simulink model "rsim_param_tuning"  (Simulink 5.0)
settings: Solver=VariableStepDiscrete  StartTime=0.0  StopTime=48  FixedStep=1  RelTol=1e-3
PreLoadFcn:
  | clear;INC=uint8(1);LIMIT=uint8(16);K=int32(2);RESET=uint8(0);
StartFcn:
  | platform_finder('')
settings Model: CovMetricSettings=d  Creator=pszpak  LastModifiedBy=dcabral  ExtModeTrigMode=oneshot  ExtModeArmWhenConnect=off  ExtModeAutoUpdateStatusClock=off  TunableVars=INC,LIMIT,RESET,K  TunableVarsStorageClass=ExportedGlobal,ExportedGlobal,ExportedGlobal,ExportedGlobal  TunableVarsTypeQualifier=,,,  BufferReuse=off  SaveFormat=StructureWithTime  LimitDataPoints=off  IntegerOverflowMsg=none  RTWInlineParameters=on  ProdHWWordLengths=8,32,16,32  RTWSystemTargetFile=rsim.tlc  RTWTemplateMakefile=rsim_default_tmf  RTWRetainRTWFile=on  RTWOptions="-aEnforceIntegerDowncast=0 -aExtMode=0 -aExtModeTesting=0 -aFoldNonRolledExpr=1 -aForceParamTrailComments=0 -aGenerateComments=1 -aGenerateReport=0 -aIncDataTypeInIds=0 -aIncHierarchyInIds=0 -aInlineInvariantSignals=1 -aInlineParameters=1 -aInlinedPrmAccess=\"Literals\" -aLocalBlockOutputs=1 -aMaxRTWIdLen=31 -aPrefixModelToSubsysFcnNames=1 -aRSIM_SOLVER_SELECTION=1 -aRTWVerbose=1 -aRollThreshold=5 -aShowEliminatedStatements=1"

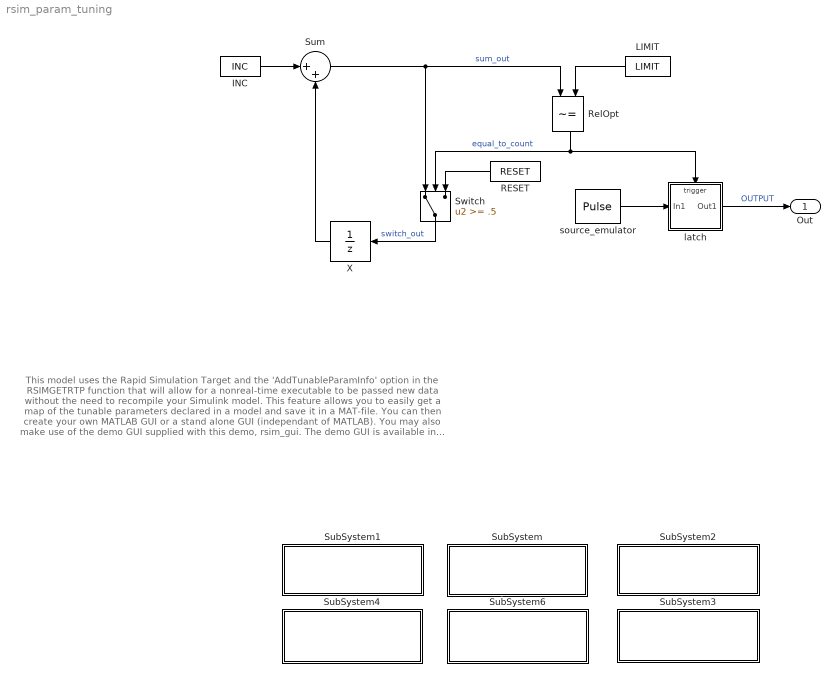
== system rsim_param_tuning ==
  note: This model uses the Rapid Simulation Target and the 'AddTunableParamInfo' option in
      | the RSIMGETRTP function that will allow for a nonreal-time executable to be passed new
      | data without the need to recompile your Simulink model. This feature allows you to easily
      | get a map of the tunable parameters declared in a model and save it in a MAT-file. You
      | can then create your own MATLAB GUI or a stand alone GUI (independant of MATLAB).
      | You may also make use of the demo GUI supplied with this demo, rsim_gui.
      |
      | The demo GUI is available in MATLAB and stand alone mode (independant of MATLAB).
      |
      | Double-click on the buttons below sequentially to run the demo. For more information on
      | the Rapid Simulation Target and to review the code used to create the both the MATLAB GUI
      | and standalone GUI, double-click on the 'More Info' button.
      |
      | For more information, you may also refer to the "Rapid Simulation Target" chapter in the
      | Real-Time Workshop User's Guide.
  INC : Constant  Value=INC
  LIMIT : Constant  Orientation=left  Value=LIMIT
  RESET : Constant  Orientation=left  Value=RESET
  RelOpt : RelationalOperator  Orientation=down  Operator=~=  InputSameDT=on
  SubSystem : Subsystem  Orientation=left
      settings: AttributesFormatString=\n\n\n\n\n\n\n\n\n
      settings: OpenFcn=|
      | disp(' ')
      | disp('% ----- STEP 2 : Running the RSIMGETRTP command ----- %')
      | disp('>>rtp=rsimgetrtp(''rsim_param_tuning'',''AddTunableParamInfo'',''on'')')
      | rtp=rsimgetrtp('rsim_param_tuning','AddTunableParamInfo','on')
      | disp('% ----- Notice the ''map'' field of the structure ----- %')
      | disp('>>rtp.parameters')
      | rtp.parameters
      | disp('% ----- Here are the contents of the ''map'' field for the first parameter ----- %')
      | disp('>>rtp.parameters(1).map(1)')
      | rtp.parameters(1).map(1)
      mask Display: disp('2. Run RSIMGETRTP\nwith the option')
  SubSystem1 : Subsystem  Orientation=left
      settings: AttributesFormatString=\n\n\n\n\n\n\n\n
      settings: OpenFcn=|
      | platform_finder('')
      | disp('% ----- STEP 1: Building the Model with Real-Time Workshop ----- %')
      | rtwbuild('rsim_param_tuning');
      mask Display: disp('1. Build Model with \n RSim Target')
  SubSystem2 : Subsystem  Orientation=left
      settings: AttributesFormatString=\n\n\n\n\n\n\n\n\n
      settings: OpenFcn=|
      | platform_finder('')
      | disp('% ----- STEP 3: Saving the rtp Structure in a MAT-File ----- %')
      | disp('>>save rsim_rtp_struct rtp')
      | save rsim_rtp_struct rtp
      mask Display: disp('3. Save RTP structure \n in a MAT-File')
  SubSystem3 : Subsystem  Orientation=left
      settings: AttributesFormatString=\n\n
      settings: OpenFcn=|
      | edit('rsim_gui.m')
      | edit('rsim_gui_sa.m')
      | edit('rtwtargetsrsim.txt')
      mask Display: disp('More Info')
  SubSystem4 : Subsystem  Orientation=left
      settings: AttributesFormatString=\n\n\n\n\n\n\n\n
      settings: OpenFcn=|
      | disp(' ')
      | platform_finder('matlab_gui')
      mask Display: disp('4. Open the MATLAB \n RSIM GUI Demo')
  SubSystem6 : Subsystem  Orientation=left
      settings: AttributesFormatString=\n\n\n\n\n\n\n\n\n
      settings: OpenFcn=|
      | disp(' ')
      | platform_finder('standalone_gui')
      mask Display: disp('Open the Standalone \n RSIM GUI Demo')
  Sum : Sum  Inputs=|++  InputSameDT=on
  Switch : Switch  Orientation=down  Threshold=.5  InputSameDT=on
  X : UnitDelay  Orientation=left  StateIdentifier=X
      settings: RTWStateStorageClass=ExportedGlobal
  latch : Subsystem  TreatAsAtomicUnit=on
  source_emulator : DiscretePulseGenerator  Amplitude=int32(1)  Period=4  PulseWidth=2
  Out : Outport
  wires:
  INC/1 -> Sum/1
  X/1 -> Sum/2
  Switch/1 -> X/1  "switch_out"
  Sum/1 -> Switch/1, RelOpt/1  "sum_out"
  LIMIT/1 -> RelOpt/2
  RESET/1 -> Switch/3
  RelOpt/1 -> latch/Trigger, Switch/2  "equal_to_count"
  latch/1(Out1) -> Out/1  "OUTPUT"
  source_emulator/1 -> latch/1(In1)

== system rsim_param_tuning/SubSystem ==

== system rsim_param_tuning/SubSystem1 ==

== system rsim_param_tuning/SubSystem2 ==

== system rsim_param_tuning/SubSystem3 ==

== system rsim_param_tuning/SubSystem4 ==

== system rsim_param_tuning/SubSystem6 ==

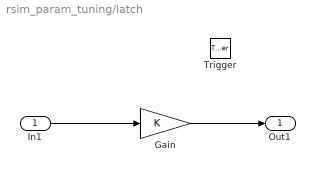
== system rsim_param_tuning/latch ==
  In1 : Inport
  Trigger : TriggerPort  ZeroCross=off
  Gain : Gain  Gain=K
  Out1 : Outport  InitialOutput=0
  wires:
  In1/1 -> Gain/1
  Gain/1 -> Out1/1
